simulink model "Two_phase_mode_inverter"  (Simulink 8.6)
settings: Solver=ode8  StartTime=0.0  StopTime=100e-3  FixedStep=1e-6  RelTol=1e-5
libraries: powerlib x19, simulink x1
settings Model: Creator=CHAMARTHI  LastModifiedBy=CHAMARTHI  PauseTimes=10e-3  NumberOfSteps=100
settings DataIOCC: SaveFormat=Dataset  SignalLoggingSaveFormat=Dataset
settings OptimizationCC: ExpressionDepthLimit=128
settings DebuggingCC: UnderspecifiedInitializationDetection=Simplified  MergeDetectMultiDrivingBlocksExec=error  SolverPrmCheckMsg=none  FcnCallInpInsideContextMsg=EnableAllAsError  StateNameClashWarn=none
settings HardwareCC: ProdBitPerPointer=64  ProdLargestAtomicFloat=Float  ProdIntDivRoundTo=Zero  ProdEndianess=LittleEndian  ProdWordSize=64  ProdHWDeviceType=Intel->x86-64 (Windows64)
settings GRTTargetCC: GeneratePreprocessorConditionals=Use local settings  CombineOutputUpdateFcns=on  GRTInterface=off
settings ConfigComp: CovModelRefEnable=off

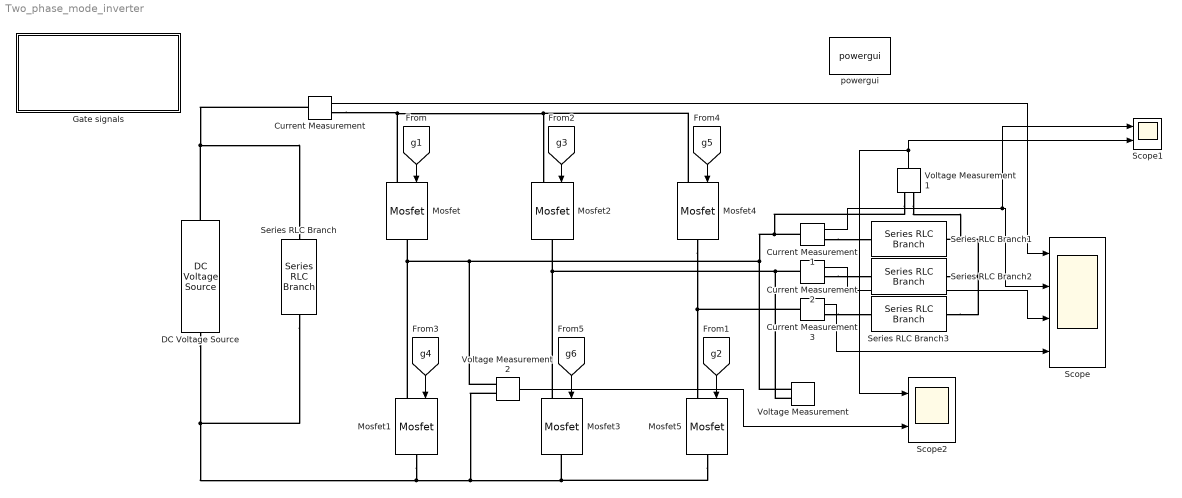
== system Two_phase_mode_inverter ==
  Current Measurement{,1..3} (4 alike) : powerlib/Measurements/Current Measurement  PhasorSimulation=off  OutputType=Complex  PSBequivalent=0
  DC Voltage Source : powerlib/Electrical Sources/DC Voltage Source  Amplitude=100  Measurements=None
  Gate signals : Subsystem
  Mosfet : powerlib/Power Electronics/Mosfet  Ron=0.01  Lon=0  Rd=0.01  Vfd=0  IC=0  Rs=1e5  Cs=inf  Measurements=off
  Mosfet1 : powerlib/Power Electronics/Mosfet  Ron=0.01  Lon=0  Rd=0.01  Vfd=0  IC=0  Rs=1e5  Cs=100e-9  Measurements=off
  Mosfet2 : powerlib/Power Electronics/Mosfet  Ron=0.01  Lon=0  Rd=0.01  Vfd=0  IC=0  Rs=1e5  Cs=inf  Measurements=off
  Mosfet3 : powerlib/Power Electronics/Mosfet  Ron=0.01  Lon=0  Rd=0.01  Vfd=0  IC=0  Rs=1e5  Cs=100e-9  Measurements=off
  Mosfet4 : powerlib/Power Electronics/Mosfet  Ron=0.01  Lon=0  Rd=0.01  Vfd=0  IC=0  Rs=1e5  Cs=inf  Measurements=off
  Mosfet5 : powerlib/Power Electronics/Mosfet  Ron=0.01  Lon=0  Rd=0.01  Vfd=0  IC=0  Rs=1e5  Cs=100e-9  Measurements=off
  Scope : Scope  NumInputPorts=4
  Scope1 : Scope  NumInputPorts=2
  Scope2 : Scope  NumInputPorts=2
  Series RLC Branch : powerlib/Elements/Series RLC Branch  LConnTagsString=__new0  RConnTagsString=__new0  BranchType=RC  Resistance=0.01  Inductance=1e-3  SetiL0=off  InitialCurrent=0  Capacitance=470e-6  Setx0=off  InitialVoltage=0  Measurements=None
  Series RLC Branch1 : powerlib/Elements/Series RLC Branch  LConnTagsString=__new0  RConnTagsString=__new0  BranchType=RL  Resistance=1  Inductance=300e-6  SetiL0=off  InitialCurrent=0  Capacitance=1e-6  Setx0=off  InitialVoltage=0  Measurements=None
  Series RLC Branch2 : powerlib/Elements/Series RLC Branch  LConnTagsString=__new0  RConnTagsString=__new0  BranchType=RL  Resistance=1  Inductance=300e-6  SetiL0=off  InitialCurrent=0  Capacitance=1e-6  Setx0=off  InitialVoltage=0  Measurements=None
  Series RLC Branch3 : powerlib/Elements/Series RLC Branch  LConnTagsString=__new0  RConnTagsString=__new0  BranchType=RL  Resistance=1  Inductance=300e-6  SetiL0=off  InitialCurrent=0  Capacitance=1e-6  Setx0=off  InitialVoltage=0  Measurements=None
  Voltage Measurement : powerlib/Measurements/Voltage Measurement  PhasorSimulation=off  OutputType=Complex  PSBequivalent=0
  Voltage Measurement1 : powerlib/Measurements/Voltage Measurement  PhasorSimulation=off  OutputType=Complex  PSBequivalent=0
  Voltage Measurement2 : powerlib/Measurements/Voltage Measurement  PhasorSimulation=off  OutputType=Complex  PSBequivalent=0
  powergui : powerlib/powergui  Priority=1  SimulationMode=Discrete  SolverType=Tustin/Backward Euler (TBE)  SampleTime=1e-6  frequency=60  SPID=off  DisableSnubberDevices=off  DisableRonSwitches=off  DisableVfSwitches=off  SwTol=0  DisplayEquations=off  Interpol=off  ExternalGateDelay=off  methode=off  Ts=10  FunctionMessages=off  echomessages=off  HookPort=off  EnableUseOfTLC=off  x0status=blocks  frequencyindice=0  Pbase=100e6  ErrMax=1e-4  Iterations=50  UnitsV=kV  UnitsW=MW  buscounter=0  RestoreLinks=warning  ResistiveCurrentMeasurement=off  Frange=[0:2:500]  Ylog=off  Xlog=on  ShowGrid=off  save=off  variable=ZData  structure=0  ZoomFFT=off  StartTime=0.0  cycles=1  DisplayStyle=1  fundamental=60  FreqAxis=off  MaxFrequency=1000  frequencyindicesteady=1  RmsSteady=1  display=off
  wires:
  [g1] -> Mosfet/1
  [g2] -> Mosfet5/1
  [g3] -> Mosfet2/1
  [g4] -> Mosfet1/1
  [g5] -> Mosfet4/1
  [g6] -> Mosfet3/1
  Current Measurement1/1 -> Scope1/1, Scope/2
  Current Measurement/1 -> Scope/1
  Current Measurement2/1 -> Scope/3
  Current Measurement3/1 -> Scope/4
  Voltage Measurement1/1 -> Scope2/1, Scope1/2
  Voltage Measurement2/1 -> Scope2/2
  connections:
  Mosfet4/RConn1 -- Current Measurement3/LConn1 -- Mosfet5/LConn1
  Mosfet3/LConn1 -- Voltage Measurement/LConn2 -- Current Measurement2/LConn1 -- Mosfet2/RConn1
  Mosfet1/LConn1 -- Voltage Measurement2/LConn1 -- Voltage Measurement/LConn1 -- Current Measurement1/LConn1 -- Voltage Measurement1/LConn1 -- Mosfet/RConn1
  Mosfet1/RConn1 -- Series RLC Branch/RConn1 -- DC Voltage Source/LConn1 -- Voltage Measurement2/LConn2 -- Mosfet3/RConn1 -- Mosfet5/RConn1
  DC Voltage Source/RConn1 -- Current Measurement/LConn1 -- Series RLC Branch/LConn1
  Series RLC Branch3/RConn1 -- Series RLC Branch2/RConn1 -- Voltage Measurement1/LConn2 -- Series RLC Branch1/RConn1
  Mosfet4/LConn1 -- Current Measurement/RConn1 -- Mosfet/LConn1 -- Mosfet2/LConn1
  Current Measurement1/RConn1 -- Series RLC Branch1/LConn1
  Current Measurement2/RConn1 -- Series RLC Branch2/LConn1
  Current Measurement3/RConn1 -- Series RLC Branch3/LConn1

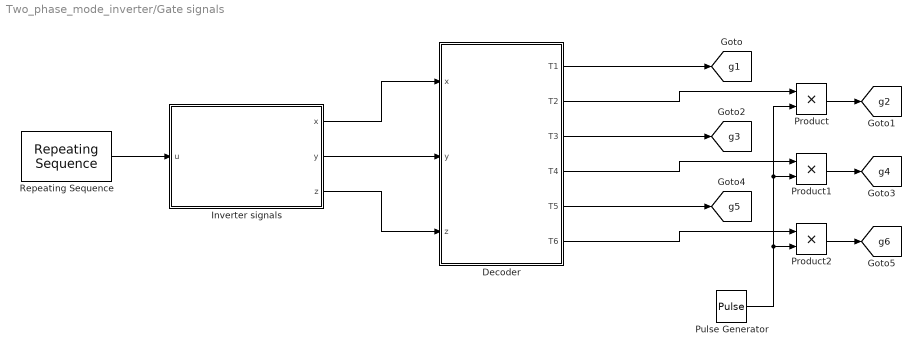
== system Two_phase_mode_inverter/Gate signals ==
  Decoder : MATLAB Function  TreatAsAtomicUnit=on
  Inverter signals : MATLAB Function  TreatAsAtomicUnit=on
  Product : Product
  Product1 : Product
  Product2 : Product
  Pulse Generator : DiscretePulseGenerator  PulseType=Time based  Period=100e-6  PulseWidth=50
  Repeating Sequence : simulink/Sources/Repeating Sequence  rep_seq_t=[0 10e-3]  rep_seq_y=[0 10]
  tag scope: g1=global, g2=global, g3=global, g4=global, g5=global, g6=global
  wires:
  Decoder/1(T1) -> [g1]
  Decoder/3(T3) -> [g3]
  Inverter signals/3(z) -> Decoder/3(z)
  Inverter signals/1(x) -> Decoder/1(x)
  Inverter signals/2(y) -> Decoder/2(y)
  Decoder/5(T5) -> [g5]
  Repeating Sequence/1 -> Inverter signals/1(u)
  Product/1 -> [g2]
  Product2/1 -> [g6]
  Product1/1 -> [g4]
  Decoder/4(T4) -> Product1/1
  Decoder/2(T2) -> Product/1
  Decoder/6(T6) -> Product2/1
  Pulse Generator/1 -> Product2/2, Product1/2, Product/2

== matlab function Gate signals/Decoder ==
  data: x input double; y input double; z input double; T1 output double; T2 output double; T3 output double; T4 output double; T5 output double; T6 output double
function [T1,T2,T3,T4,T5,T6] = Gate_signals(x,y,z)
T1 = 0;
T2 = 0;
T3 = 0;
T4 = 0;
T5 = 0;
T6 = 0;
if((x == 0)&&(y == 0)&&(z == 1))
    % T1 and T2 are on
    T1 = 1;
    T2 = 1;
    T3 = 0;
    T4 = 0;
    T5 = 0;
    T6 = 0;
elseif((x == 0)&&(y == 1)&&(z == 0))
    % T2 and T3 are on
    T1 = 0;
    T2 = 1;
    T3 = 1;
    T4 = 0;
    T5 = 0;
    T6 = 0;
elseif((x == 0)&&(y == 1)&&(z == 1))
    % T3 and T4 are on
    T1 = 0;
    T2 = 0;
    T3 = 1;
    T4 = 1;
    T5 = 0;
    T6 = 0;
elseif((x == 1)&&(y == 0)&&(z == 0))
    % T4 and T5 are on
    T1 = 0;
    T2 = 0;
    T3 = 0;
    T4 = 1;
    T5 = 1;
    T6 = 0;
elseif((x == 1)&&(y == 0)&&(z == 1))
    % T5 and T6 are on
    T1 = 0;
    T2 = 0;
    T3 = 0;
    T4 = 0;
    T5 = 1;
    T6 = 1;
elseif((x == 1)&&(y == 1)&&(z == 0))
    % T6 and T1 are on
    T1 = 1;
    T2 = 0;
    T3 = 0;
    T4 = 0;
    T5 = 0;
    T6 = 1;
end
end

== matlab function Gate signals/Inverter signals ==
  data: u input double; x output double; y output double; z output double
function [x,y,z] = Two_phase_mode(u)
x = 0;
y = 0;
z = 0;
if((0 <= u)&&(u < 1.6667))
    x = 0;
    y = 0;
    z = 1;
elseif((1.6667 <= u)&&(u < 3.3333))
    x = 0;
    y = 1;
    z = 0;
elseif((3.3333 <= u)&&(u < 5))
    x = 0;
    y = 1;
    z = 1;
elseif((5 <= u)&&(u < 6.6667))
    x = 1;
    y = 0;
    z = 0;
elseif((6.6667 <= u)&&(u < 8.3333))
    x = 1;
    y = 0;
    z = 1;
elseif((8.3333 <= u)&&(u < 10))
    x = 1;
    y = 1;
    z = 0;
end
end
